simulink subsystem "HeadingRateController"  (R2022b)
settings: Solver=VariableStepAuto  StartTime=0.0  StopTime=10.0  RelTol=1e-3
settings Model: Creator=Sahil Gaurkar  LastModifiedBy=Wikian

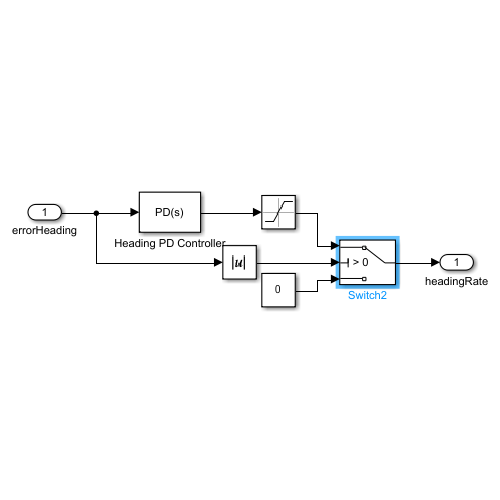
[thumbnail: Simulink's stored preview of the top-level diagram]
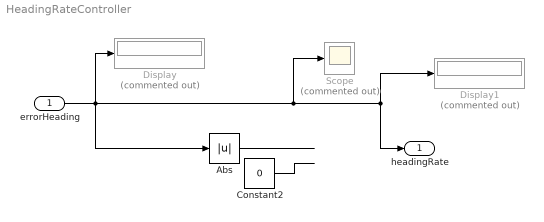
== system HeadingRateController ==
  errorHeading : Inport
  Abs : Abs  SaturateOnIntegerOverflow=off
  Constant2 : Constant  Value=0
  Display : Display  Commented=on
  Display1 : Display  Commented=on
  Scope : Scope  Commented=on
  headingRate : Outport
  wires:
  Abs/1 -> ?
  errorHeading/1 -> Display/1, Abs/1, Scope/1, Display1/1, headingRate/1
  Constant2/1 -> ?
